simulink model "DCM2Euler_Test_Sim"  (Simulink 7.5)
settings: Solver=ode45  StartTime=0.0  StopTime=10.0  RelTol=1e-3
libraries: SLUGS_Library x3, simulink x1
settings Model: Creator=Robert  LastModifiedBy=Robert

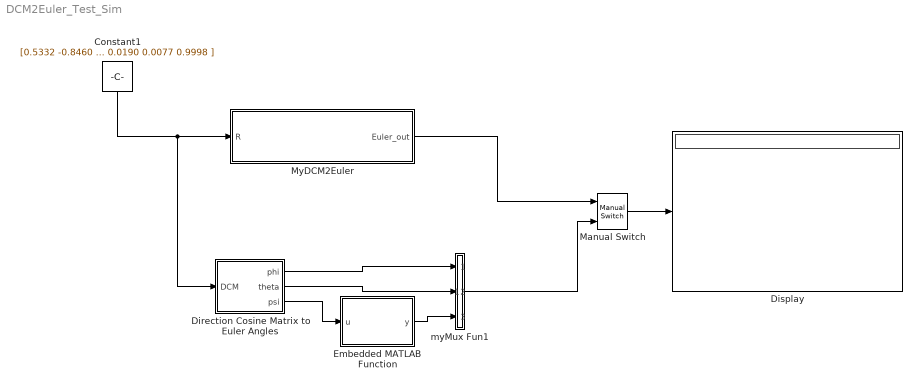
== system DCM2Euler_Test_Sim ==
  Constant1 : Constant  Value=[0.5332 -0.8460 -0.0036; 0.8458 0.5332 -0.0202; 0.0190 0.0077 0.9998 ]  VectorParams1D=off  OutDataTypeMode=single  OutDataType=sfix(16)  OutScaling=2^0  OutDataTypeStr=single
  Direction Cosine Matrix to Euler Angles : Subsystem  AncestorBlock=aerolibtransform2/Direction Cosine Matrix to Euler Angles  mask(DCM2Euler){}
      mask help: Determine an euler orientation (roll, pitch, yaw) from the 3-by-3 direction cosine matrix (DCM). The input DCM transforms vectors from geodetic earth or north-down-east (NED) axes to body axes.
      mask init:
      | aeroicon('aeroblk');
      mask Help: web(asbhelp('directioncosinematrixtoeulerangles'));
      mask Display:
      | port_label('output',1,'\phi','texmode','on')
      | port_label('output',2,'\theta','texmode','on')
      | port_label('output',3,'\psi','texmode','on')
      | port_label('input',1,'DCM_{be}','texmode','on')
  Display : Display
  Embedded MATLAB Function : Stateflow chart  TreatAsAtomicUnit=on
  Manual Switch : simulink/Signal Routing/Manual Switch  SystemSampleTime=-1  sw=0  action=0  varsize=off
  MyDCM2Euler : Stateflow chart  TreatAsAtomicUnit=on
  myMux Fun1 : Stateflow chart  TreatAsAtomicUnit=on
  wires:
  Constant1/1 -> MyDCM2Euler/1(R), Direction Cosine Matrix to Euler Angles/1(DCM)
  Embedded MATLAB Function/1(y) -> myMux Fun1/3(u3)
  Direction Cosine Matrix to Euler Angles/2(theta) -> myMux Fun1/2(u2)
  Direction Cosine Matrix to Euler Angles/1(phi) -> myMux Fun1/1(u1)
  Direction Cosine Matrix to Euler Angles/3(psi) -> Embedded MATLAB Function/1(u)
  myMux Fun1/1(y) -> Manual Switch/2
  Manual Switch/1 -> Display/1
  MyDCM2Euler/1(Euler_out) -> Manual Switch/1

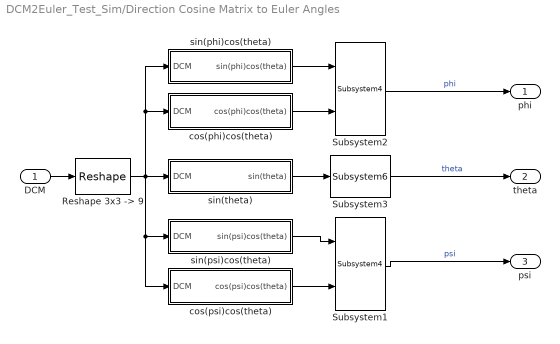
== system DCM2Euler_Test_Sim/Direction Cosine Matrix to Euler Angles ==
  DCM : Inport  PortDimensions=[3,3]  OutDataType=sfix(16)  OutScaling=2^0
  "Reshape 3x3 -> 9" : Reshape  OutputDimensions=[9, 1]
  Subsystem1 : SLUGS_Library/Subsystem4  SystemSampleTime=-1
  Subsystem2 : SLUGS_Library/Subsystem4  SystemSampleTime=-1
  Subsystem3 : SLUGS_Library/Subsystem6  SystemSampleTime=-1
  cos(phi)cos(theta) : Subsystem
  cos(psi)cos(theta) : Subsystem
  sin(phi)cos(theta) : Subsystem
  sin(psi)cos(theta) : Subsystem
  sin(theta) : Subsystem
  phi : Outport  PortDimensions=1  OutDataType=sfix(16)  OutScaling=2^0  InitialOutput=0
  theta : Outport  Port=2  PortDimensions=1  OutDataType=sfix(16)  OutScaling=2^0  InitialOutput=0
  psi : Outport  Port=3  PortDimensions=1  OutDataType=sfix(16)  OutScaling=2^0  InitialOutput=0
  wires:
  DCM/1 -> "Reshape 3x3 -> 9"/1
  "Reshape 3x3 -> 9"/1 -> sin(theta)/1(DCM), cos(phi)cos(theta)/1(DCM), sin(phi)cos(theta)/1(DCM), cos(psi)cos(theta)/1(DCM), sin(psi)cos(theta)/1(DCM)
  sin(theta)/1(sin(theta)) -> Subsystem3/1
  sin(phi)cos(theta)/1(sin(phi)cos(theta)) -> Subsystem2/1
  cos(phi)cos(theta)/1(cos(phi)cos(theta)) -> Subsystem2/2
  sin(psi)cos(theta)/1(sin(psi)cos(theta)) -> Subsystem1/1
  cos(psi)cos(theta)/1(cos(psi)cos(theta)) -> Subsystem1/2
  Subsystem2/1 -> phi/1  "phi"
  Subsystem3/1 -> theta/1  "theta"
  Subsystem1/1 -> psi/1  "psi"

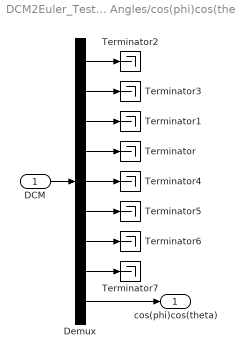
== system DCM2Euler_Test_Sim/Direction Cosine Matrix to Euler Angles/cos(phi)cos(theta) ==
  DCM : Inport  OutDataType=sfix(16)  OutScaling=2^0
  Demux : Demux  Outputs=9
  Terminator{,1..7} (8 alike) : Terminator
  cos(phi)cos(theta) : Outport  OutDataType=sfix(16)  OutScaling=2^0
  wires:
  Demux/4 -> Terminator/1
  Demux/3 -> Terminator1/1
  Demux/5 -> Terminator4/1
  Demux/2 -> Terminator3/1
  Demux/1 -> Terminator2/1
  DCM/1 -> Demux/1
  Demux/8 -> Terminator7/1
  Demux/6 -> Terminator5/1
  Demux/7 -> Terminator6/1
  Demux/9 -> cos(phi)cos(theta)/1

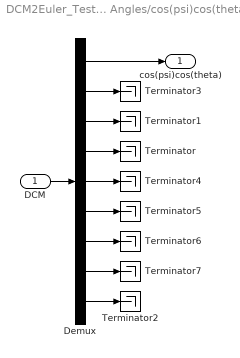
== system DCM2Euler_Test_Sim/Direction Cosine Matrix to Euler Angles/cos(psi)cos(theta) ==
  DCM : Inport  OutDataType=sfix(16)  OutScaling=2^0
  Demux : Demux  Outputs=9
  Terminator{,1..7} (8 alike) : Terminator
  cos(psi)cos(theta) : Outport  OutDataType=sfix(16)  OutScaling=2^0
  wires:
  Demux/9 -> Terminator2/1
  Demux/7 -> Terminator6/1
  Demux/6 -> Terminator5/1
  Demux/8 -> Terminator7/1
  DCM/1 -> Demux/1
  Demux/1 -> cos(psi)cos(theta)/1
  Demux/2 -> Terminator3/1
  Demux/5 -> Terminator4/1
  Demux/3 -> Terminator1/1
  Demux/4 -> Terminator/1

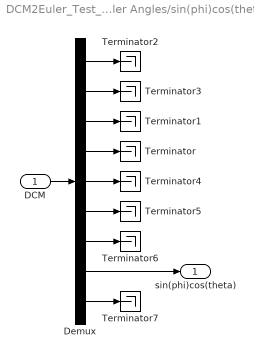
== system DCM2Euler_Test_Sim/Direction Cosine Matrix to Euler Angles/sin(phi)cos(theta) ==
  DCM : Inport  OutDataType=sfix(16)  OutScaling=2^0
  Demux : Demux  Outputs=9
  Terminator{,1..7} (8 alike) : Terminator
  sin(phi)cos(theta) : Outport  OutDataType=sfix(16)  OutScaling=2^0
  wires:
  Demux/9 -> Terminator7/1
  Demux/7 -> Terminator6/1
  Demux/6 -> Terminator5/1
  Demux/8 -> sin(phi)cos(theta)/1
  DCM/1 -> Demux/1
  Demux/1 -> Terminator2/1
  Demux/2 -> Terminator3/1
  Demux/5 -> Terminator4/1
  Demux/3 -> Terminator1/1
  Demux/4 -> Terminator/1

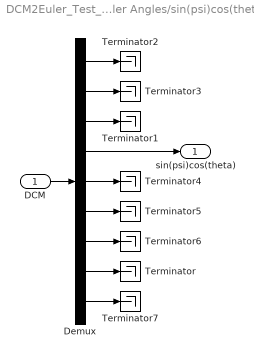
== system DCM2Euler_Test_Sim/Direction Cosine Matrix to Euler Angles/sin(psi)cos(theta) ==
  DCM : Inport  OutDataType=sfix(16)  OutScaling=2^0
  Demux : Demux  Outputs=9
  Terminator{,1..7} (8 alike) : Terminator
  sin(psi)cos(theta) : Outport  OutDataType=sfix(16)  OutScaling=2^0
  wires:
  Demux/4 -> sin(psi)cos(theta)/1
  Demux/3 -> Terminator1/1
  Demux/5 -> Terminator4/1
  Demux/2 -> Terminator3/1
  Demux/1 -> Terminator2/1
  DCM/1 -> Demux/1
  Demux/8 -> Terminator/1
  Demux/6 -> Terminator5/1
  Demux/7 -> Terminator6/1
  Demux/9 -> Terminator7/1

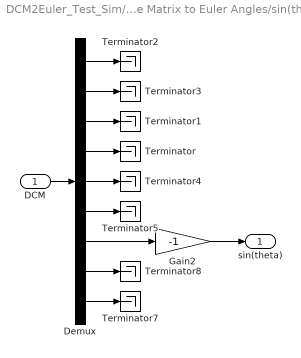
== system DCM2Euler_Test_Sim/Direction Cosine Matrix to Euler Angles/sin(theta) ==
  DCM : Inport  OutDataType=sfix(16)  OutScaling=2^0
  Demux : Demux  Outputs=9
  Gain2 : Gain  Gain=-1  ParameterDataType=sfix(16)  ParameterScaling=2^0  OutDataType=sfix(16)  OutScaling=2^0  SaturateOnIntegerOverflow=on  OutDataTypeStr=Inherit: Same as input  ParamDataTypeStr=Inherit: Same as input
  Terminator{,1..5,7..8} (8 alike) : Terminator
  sin(theta) : Outport  OutDataType=sfix(16)  OutScaling=2^0
  wires:
  Gain2/1 -> sin(theta)/1
  Demux/4 -> Terminator/1
  Demux/3 -> Terminator1/1
  Demux/5 -> Terminator4/1
  Demux/2 -> Terminator3/1
  Demux/1 -> Terminator2/1
  DCM/1 -> Demux/1
  Demux/8 -> Terminator8/1
  Demux/6 -> Terminator5/1
  Demux/7 -> Gain2/1
  Demux/9 -> Terminator7/1

== matlab function Embedded MATLAB Function ==
  data: u input double; y output double
function y = TwoPi(u)
% This block supports an embeddable subset of the MATLAB language.
% See the help menu for details. 

if ( u < 0 )
    y = u + 2*pi;
else
    y = u;
end

== matlab function myMux Fun1 ==
  data: u1 input double; y output double; u2 input double; u3 input double
function y = myMux3(u1, u2, u3)
% This block supports an embeddable subset of the MATLAB language.
% See the help menu for details. 

y = [u1(1); u2(1); u3(1)];

== matlab function MyDCM2Euler ==
  data: R input double; Euler_out output double
function Euler_out  = MyDCM2Euler( R )
%#eml
%DCM2EULER Function converts a Direction Cosine Matrix into 
%   its corresponding 3-2-1 Euler angle parameterization.
%   PARAMETERS
%   R = input DCM, 3x3 matrix
%   RETVAL
%   Euler_out = output Euler angles in a column vector (3x1), radians
    Euler_out = single( zeros( 3, 1 ) );
    Euler_out( 1 ) = atan2( R( 3, 2 ), R( 3, 3 ));  % phi
    Euler_out( 2 ) = -asin( R( 3, 1 ));             % theta
    Euler_out( 3 ) = atan2( R( 2, 1 ), R( 1, 1 ));  % psi
    % 10/22/12 edit - no negative yaw/psi
    if( Euler_out(3) < 0 )
        Euler_out(3) = Euler_out(3) + 2 * pi;
    end
end
